simulink model "manufacturing_cell"  (R2026a)
settings: Solver=VariableStepAuto  StopTime=1000
undefined symbols (not defined in the file): m, n
settings Model: Creator=soumy  LastModifiedBy=soumy

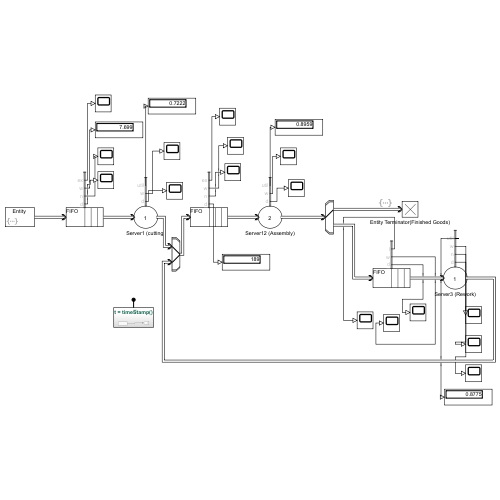
[thumbnail: Simulink's stored preview of the top-level diagram]
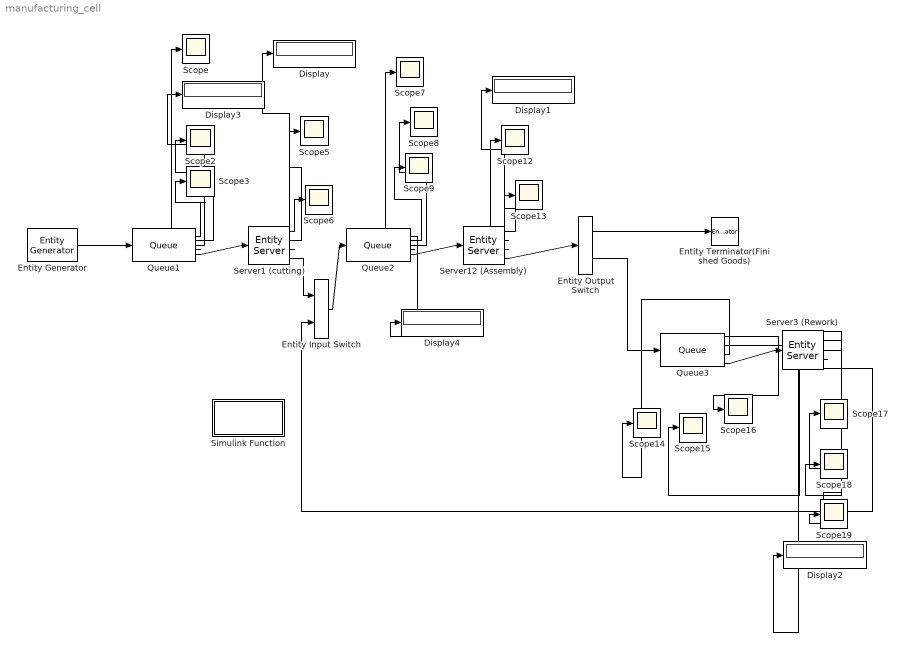
== system manufacturing_cell ==
  Display{,1..4} (5 alike) : Display
  Entity Input Switch : EntityInputSwitch  InputPortMessageModes=m,m  OutputPortMessageModes=m
  Entity Output Switch : EntityOutputSwitch  InputPortMessageModes=m  OutputPortMessageModes=m,m  SwitchingCriterion=From attribute  SwitchAttributeName=Attribute1
  Entity Generator : EntityGenerator  OutputPortMessageModes=m  TimeSource=MATLAB action  Period=5  IntergenerationTimeAction=dt = -5*log(rand);  GenerateAction=|  AttributeName=Attribute1|genTime  AttributeInitialValue=1|0  EntityType=Structured  EntityTypeName=Entity
      | entity.Attribute1 = (rand() > 0.85) + 1;
      | entity.genTime = timeStamp();
  Entity Terminator(Finished Goods) : EntityTerminator  InputPortMessageModes=m  EntryAction=|
      | persistent cycleTimes
      | if isempty(cycleTimes)
      |     cycleTimes = [];
      | end
      | ct = timeStamp() - entity.genTime;
      | cycleTimes(end+1) = ct;
      | assignin('base', 'cycleTimes', cycleTimes);
  Queue1 : Queue  InputPortMessageModes=m  OutputPortMessageModes=n,n,n,n,m  Capacity=10  NumberEntitiesDeparted=on  NumEntitiesExtracted=on  NumberEntitiesInBlock=on  AverageWait=on
      settings: OutputPortMap=o0,o1,o2,o7,o5
  Queue2 : Queue  InputPortMessageModes=m  OutputPortMessageModes=n,n,n,n,m  Capacity=10  NumberEntitiesDeparted=on  NumEntitiesExtracted=on  NumberEntitiesInBlock=on  AverageWait=on
      settings: OutputPortMap=o0,o1,o2,o7,o5
  Queue3 : Queue  InputPortMessageModes=m  OutputPortMessageModes=n,n,n,m  Capacity=10  NumberEntitiesDeparted=on  AverageWait=on  AverageQueueLength=on
      settings: OutputPortMap=o0,o2,o3,o5
  Scope{,2..3,5..9,12..19} (16 alike) : Scope
      Scope12 settings: DataLoggingVariableName=ScopeData12
      Scope13 settings: DataLoggingVariableName=ScopeData13
      Scope14 settings: DataLoggingVariableName=ScopeData14
      Scope15 settings: DataLoggingVariableName=ScopeData15
      Scope16 settings: DataLoggingVariableName=ScopeData16
      Scope17 settings: DataLoggingVariableName=ScopeData17
      Scope18 settings: DataLoggingVariableName=ScopeData18
      Scope19 settings: DataLoggingVariableName=ScopeData19
      Scope2 settings: DataLoggingVariableName=ScopeData2
      Scope3 settings: DataLoggingVariableName=ScopeData3
      Scope5 settings: DataLoggingVariableName=ScopeData5
      Scope6 settings: DataLoggingVariableName=ScopeData6
      Scope7 settings: DataLoggingVariableName=ScopeData7
      Scope8 settings: DataLoggingVariableName=ScopeData8
      Scope9 settings: DataLoggingVariableName=ScopeData9
  Server1 (cutting) : EntityServer  InputPortMessageModes=m  OutputPortMessageModes=n,n,n,m  Capacity=1  ServiceTimeSource=MATLAB action  ServiceTimeAction=dt = -4*log(rand);  NumberEntitiesDeparted=on  AverageWait=on  Utilization=on
      settings: OutputPortMap=o0,o4,o5,o9
  Server12 (Assembly) : EntityServer  InputPortMessageModes=m  OutputPortMessageModes=n,n,n,m  Capacity=2  ServiceTimeSource=MATLAB action  ServiceTimeAction=dt = -6*log(rand);  NumberEntitiesDeparted=on  AverageWait=on  Utilization=on
      settings: OutputPortMap=o0,o4,o5,o9
  Server3 (Rework) : EntityServer  InputPortMessageModes=m  OutputPortMessageModes=n,n,n,n,m  Capacity=1  ServiceTimeSource=MATLAB action  ServiceTimeAction=dt = -8*log(rand);  NumberEntitiesDeparted=on  NumberEntitiesInBlock=on  AverageWait=on  Utilization=on
      settings: OutputPortMap=o0,o1,o4,o5,o9
  Simulink Function : Subsystem  TreatAsAtomicUnit=on
  wires:
  Entity Generator/1 -> Queue1/1
  Queue1/5 -> Server1 (cutting)/1
  Queue2/5 -> Server12 (Assembly)/1
  Entity Output Switch/1 -> Entity Terminator(Finished Goods)/1
  Entity Output Switch/2 -> Queue3/1
  Queue3/4 -> Server3 (Rework)/1
  Server12 (Assembly)/4 -> Entity Output Switch/1
  Queue1/4 -> Scope/1
  Queue1/3 -> Display3/1
  Queue1/2 -> Scope2/1
  Queue1/1 -> Scope3/1
  Server1 (cutting)/2 -> Scope5/1
  Server1 (cutting)/1 -> Scope6/1
  Queue2/4 -> Scope7/1
  Queue2/3 -> Scope8/1
  Queue2/2 -> Scope9/1
  Server12 (Assembly)/3 -> Display1/1
  Server12 (Assembly)/2 -> Scope12/1
  Server12 (Assembly)/1 -> Scope13/1
  Queue3/3 -> Scope14/1
  Queue3/2 -> Scope15/1
  Queue3/1 -> Scope16/1
  Server3 (Rework)/3 -> Scope17/1
  Server3 (Rework)/2 -> Scope18/1
  Server3 (Rework)/1 -> Scope19/1
  Server1 (cutting)/4 -> Entity Input Switch/1
  Entity Input Switch/1 -> Queue2/1
  Server3 (Rework)/5 -> Entity Input Switch/2
  Server1 (cutting)/3 -> Display/1
  Server3 (Rework)/4 -> Display2/1
  Queue2/1 -> Display4/1

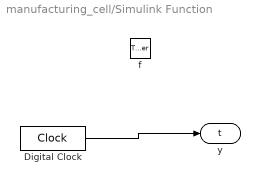
== system manufacturing_cell/Simulink Function ==
  f : TriggerPort  TriggerType=function-call  IsSimulinkFunction=on  FunctionName=timeStamp  FunctionVisibility=scoped  VariantControl=(inherit)
  Digital Clock : DigitalClock  SampleTime=-1
  y : ArgOut  DisableCoverage=on  ArgumentName=t
  wires:
  Digital Clock/1 -> y/1
